simulink model "HodHox"  (Simulink 4.00)
settings: Solver=ode45  StartTime=0.0  StopTime=15.0  RelTol=1e-3
libraries: simulink3 x1
settings Model: RTWOptions="-aExtMode=0 -aForceParamTrailComments=0 -aInlineInvariantSignals=0 -aLocalBlockOutputs=1 -aLogVarNameModifier=\"rt_\" -aRTWVerbose=1 -aRollThreshold=5 -aShowEliminatedStatements=1"  BlockReductionOpt=off

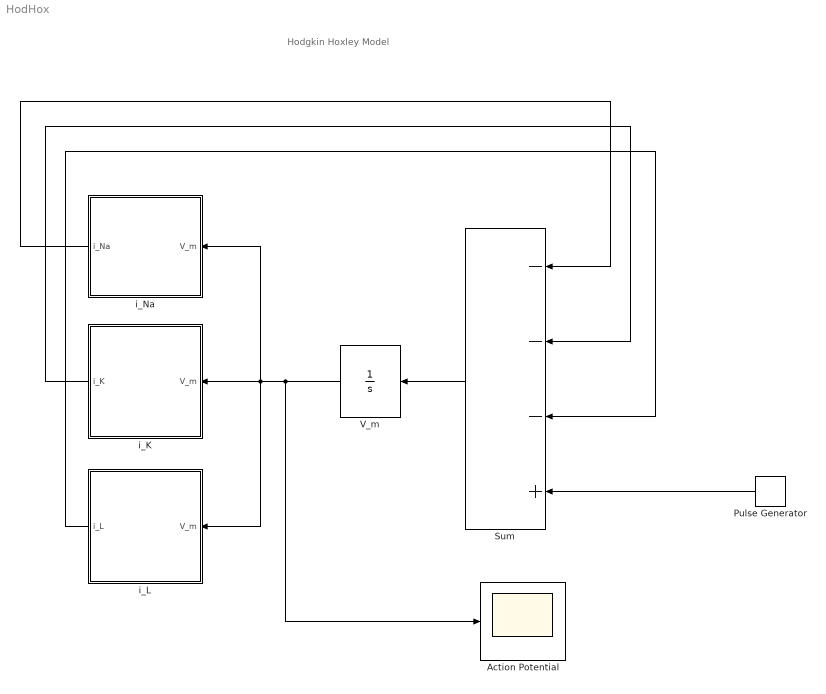
== system HodHox ==
  note: Hodgkin Hoxley Model
  Action Potential : Scope
      settings: TimeRange=10  YMin=-55  YMax=0  SaveToWorkspace=off  SaveName=ScopeData  LimitDataPoints=on  MaxDataPoints=5000
  Pulse Generator : simulink3/Sources/Pulse Generator  Orientation=left  period=2  duty=50  amplitude=15  start=5
  Sum : Sum  Orientation=left  Inputs=---+  SaturateOnIntegerOverflow=on
  V_m : Integrator  Orientation=left  ExternalReset=none  InitialConditionSource=internal  InitialCondition=0  LimitOutput=off  UpperSaturationLimit=inf  LowerSaturationLimit=-inf  ShowSaturationPort=off  ShowStatePort=off  AbsoluteTolerance=auto
  i_K : Subsystem  Orientation=left
      settings: RTWFcnNameOpts=Auto  RTWFileNameOpts=Auto
  i_L : Subsystem  Orientation=left
      settings: RTWFcnNameOpts=Auto  RTWFileNameOpts=Auto
  i_Na : Subsystem  Orientation=left
      settings: RTWFcnNameOpts=Auto  RTWFileNameOpts=Auto
  wires:
  Sum/1 -> V_m/1
  i_Na/1(i_Na) -> Sum/1
  i_K/1(i_K) -> Sum/2
  i_L/1(i_L) -> Sum/3
  Pulse Generator/1 -> Sum/4
  V_m/1 -> i_K/1(V_m), i_Na/1(V_m), i_L/1(V_m), Action Potential/1

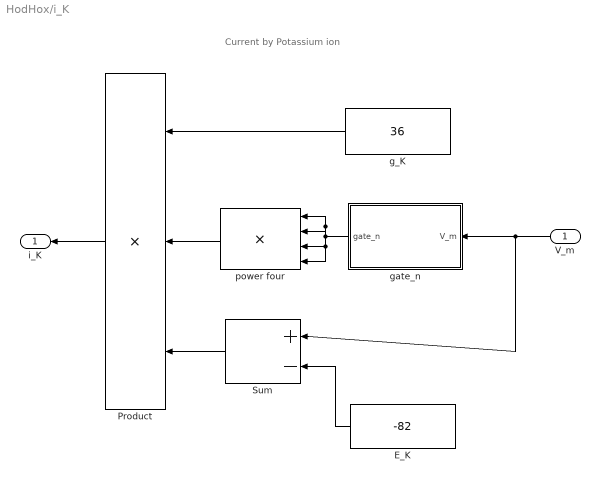
== system HodHox/i_K ==
  note: Current by Potassium ion
  V_m : Inport  Orientation=left  Port=1
  E_K : Constant  Orientation=left  Value=-82
  Product : Product  Orientation=left  Inputs=3  Multiplication=Element-wise(.*)  SaturateOnIntegerOverflow=on
  Sum : Sum  Orientation=left  Inputs=|+-  SaturateOnIntegerOverflow=on
  g_K : Constant  Orientation=left  Value=36
  gate_n : Subsystem  Orientation=left
      settings: RTWFcnNameOpts=Auto  RTWFileNameOpts=Auto
  power four : Product  Orientation=left  Inputs=4  Multiplication=Element-wise(.*)  SaturateOnIntegerOverflow=on
  i_K : Outport  Orientation=left  Port=1
  wires:
  E_K/1 -> Sum/2
  V_m/1 -> gate_n/1(V_m), Sum/1
  gate_n/1(gate_n) -> power four/4, power four/3, power four/1, power four/2
  power four/1 -> Product/2
  g_K/1 -> Product/1
  Sum/1 -> Product/3
  Product/1 -> i_K/1

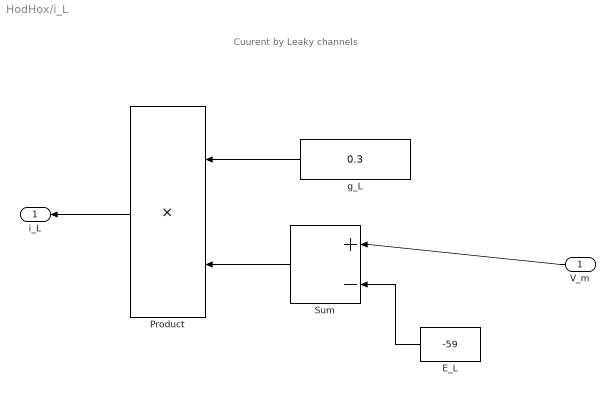
== system HodHox/i_L ==
  note: Cuurent by Leaky channels
  V_m : Inport  Orientation=left  Port=1
  E_L : Constant  Orientation=left  Value=-59
  Product : Product  Orientation=left  Inputs=2  Multiplication=Element-wise(.*)  SaturateOnIntegerOverflow=on
  Sum : Sum  Orientation=left  Inputs=|+-  SaturateOnIntegerOverflow=on
  g_L : Constant  Orientation=left  Value=0.3
  i_L : Outport  Orientation=left  Port=1
  wires:
  g_L/1 -> Product/1
  Sum/1 -> Product/2
  V_m/1 -> Sum/1
  E_L/1 -> Sum/2
  Product/1 -> i_L/1

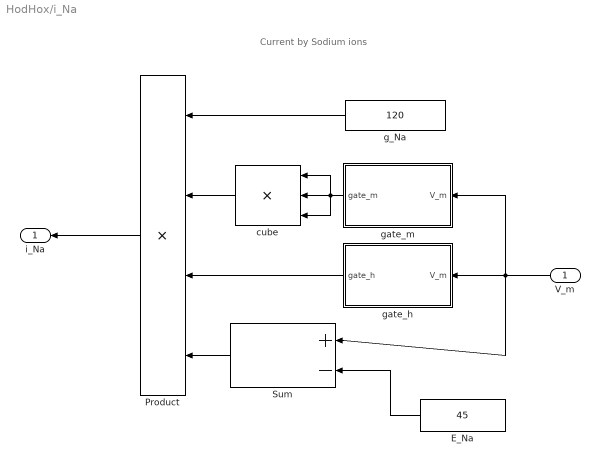
== system HodHox/i_Na ==
  note: Current by Sodium ions
  V_m : Inport  Orientation=left  Port=1
  E_Na : Constant  Orientation=left  Value=45
  Product : Product  Orientation=left  Inputs=4  Multiplication=Element-wise(.*)  SaturateOnIntegerOverflow=on
  Sum : Sum  Orientation=left  Inputs=|+-  SaturateOnIntegerOverflow=on
  cube : Product  Orientation=left  Inputs=3  Multiplication=Element-wise(.*)  SaturateOnIntegerOverflow=on
  g_Na : Constant  Orientation=left  Value=120
  gate_h : Subsystem  Orientation=left
      settings: RTWFcnNameOpts=Auto  RTWFileNameOpts=Auto
  gate_m : Subsystem  Orientation=left
      settings: RTWFcnNameOpts=Auto  RTWFileNameOpts=Auto
  i_Na : Outport  Orientation=left  Port=1
  wires:
  g_Na/1 -> Product/1
  gate_m/1(gate_m) -> cube/1, cube/3, cube/2
  cube/1 -> Product/2
  V_m/1 -> gate_m/1(V_m), gate_h/1(V_m), Sum/1
  gate_h/1(gate_h) -> Product/3
  Sum/1 -> Product/4
  E_Na/1 -> Sum/2
  Product/1 -> i_Na/1

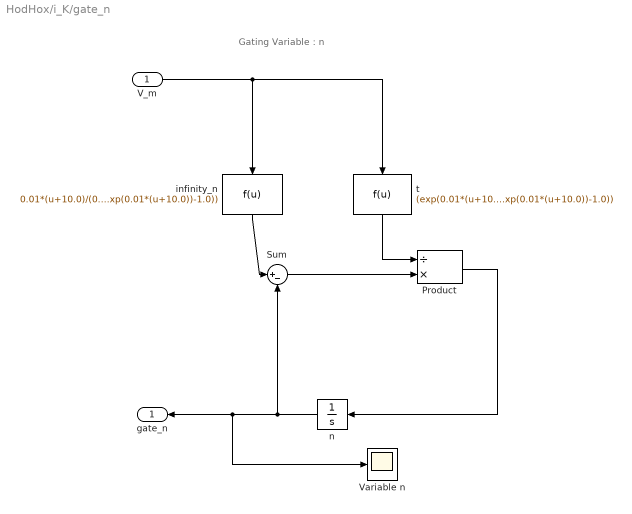
== system HodHox/i_K/gate_n ==
  note: Gating Variable : n
  V_m : Inport  Port=1
  Product : Product  Inputs=/*  Multiplication=Element-wise(.*)  SaturateOnIntegerOverflow=on
  Sum : Sum  Inputs=|+-  SaturateOnIntegerOverflow=on
  Variable n : Scope
      settings: TimeRange=auto  YMin=-5  YMax=5  SaveToWorkspace=off  SaveName=ScopeData3  LimitDataPoints=on  MaxDataPoints=5000
  infinity_n : Fcn  Orientation=down  Expr=0.01*(u+10.0)/(0.01*(u+10.0)+0.125*exp(u/80)*(exp(0.01*(u+10.0))-1.0))
  n : Integrator  Orientation=left  ExternalReset=none  InitialConditionSource=internal  InitialCondition=0  LimitOutput=off  UpperSaturationLimit=inf  LowerSaturationLimit=-inf  ShowSaturationPort=off  ShowStatePort=off  AbsoluteTolerance=auto
  t : Fcn  Orientation=down  Expr=(exp(0.01*(u+10.0))-1.0)/(0.01*(u+10.0)+0.125*exp(u/80)*(exp(0.01*(u+10.0))-1.0))
  gate_n : Outport  Orientation=left  Port=1
  wires:
  V_m/1 -> t/1, infinity_n/1
  t/1 -> Product/1
  Sum/1 -> Product/2
  infinity_n/1 -> Sum/1
  Product/1 -> n/1
  n/1 -> Sum/2, gate_n/1, Variable n/1

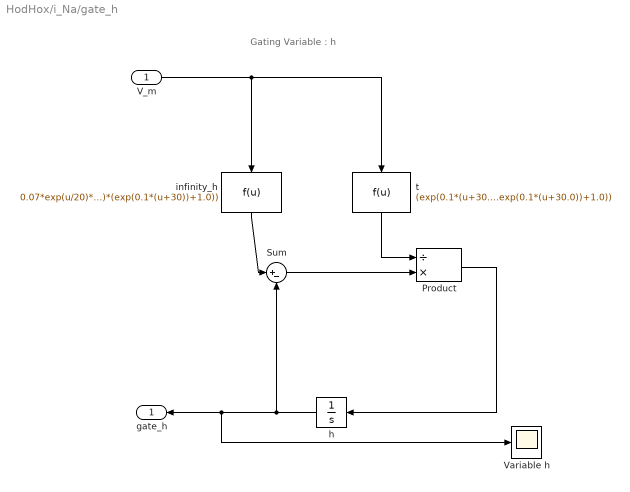
== system HodHox/i_Na/gate_h ==
  note: Gating Variable : h
  V_m : Inport  Port=1
  Product : Product  Inputs=/*  Multiplication=Element-wise(.*)  SaturateOnIntegerOverflow=on
  Sum : Sum  Inputs=|+-  SaturateOnIntegerOverflow=on
  Variable h : Scope
      settings: TimeRange=auto  YMin=-5  YMax=5  SaveToWorkspace=off  SaveName=ScopeData2  LimitDataPoints=on  MaxDataPoints=5000
  h : Integrator  Orientation=left  ExternalReset=none  InitialConditionSource=internal  InitialCondition=0  LimitOutput=off  UpperSaturationLimit=inf  LowerSaturationLimit=-inf  ShowSaturationPort=off  ShowStatePort=off  AbsoluteTolerance=auto
  infinity_h : Fcn  Orientation=down  Expr=0.07*exp(u/20)*(exp(0.1*(u+30.0))+1.0)/(1.0+0.07*exp(u/20.0)*(exp(0.1*(u+30))+1.0))
  t : Fcn  Orientation=down  Expr=(exp(0.1*(u+30.0))+1.0)/(1.0+0.07*exp(u/20.0)*(exp(0.1*(u+30.0))+1.0))
  gate_h : Outport  Orientation=left  Port=1
  wires:
  V_m/1 -> t/1, infinity_h/1
  t/1 -> Product/1
  Sum/1 -> Product/2
  infinity_h/1 -> Sum/1
  Product/1 -> h/1
  h/1 -> Sum/2, gate_h/1, Variable h/1

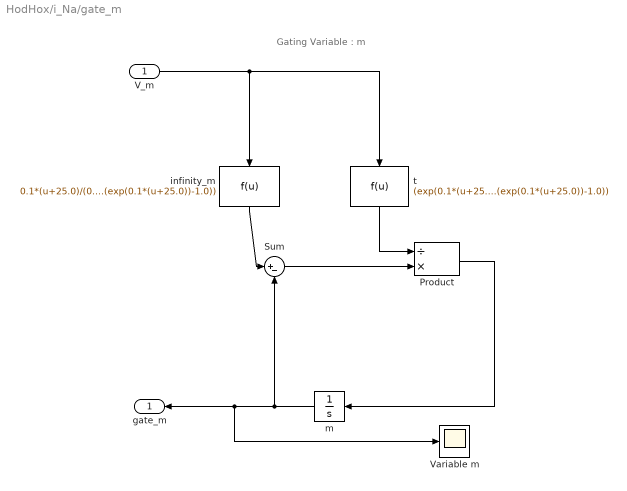
== system HodHox/i_Na/gate_m ==
  note: Gating Variable : m
  V_m : Inport  Port=1
  Product : Product  Inputs=/*  Multiplication=Element-wise(.*)  SaturateOnIntegerOverflow=on
  Sum : Sum  Inputs=|+-  SaturateOnIntegerOverflow=on
  Variable m : Scope
      settings: TimeRange=auto  YMin=-5  YMax=5  SaveToWorkspace=off  LimitDataPoints=on  MaxDataPoints=5000
  infinity_m : Fcn  Orientation=down  Expr=0.1*(u+25.0)/(0.1*(u+25.0)+4.0*(exp(u/18))*(exp(0.1*(u+25.0))-1.0))
  m : Integrator  Orientation=left  ExternalReset=none  InitialConditionSource=internal  InitialCondition=0  LimitOutput=off  UpperSaturationLimit=inf  LowerSaturationLimit=-inf  ShowSaturationPort=off  ShowStatePort=off  AbsoluteTolerance=auto
  t : Fcn  Orientation=down  Expr=(exp(0.1*(u+25.0))-1.0)/(0.1*(u+25.0)+4.0*exp(u/18.0)*(exp(0.1*(u+25.0))-1.0))
  gate_m : Outport  Orientation=left  Port=1
  wires:
  V_m/1 -> t/1, infinity_m/1
  t/1 -> Product/1
  Sum/1 -> Product/2
  infinity_m/1 -> Sum/1
  Product/1 -> m/1
  m/1 -> Sum/2, gate_m/1, Variable m/1
